simulink model "L_Trajectory_Tracking_and_Cartesian_Regulation"  (R2025b)
settings: Solver=FixedStepAuto  StartTime=0.0  StopTime=20.3895  FixedStep=Ts  RelTol=1e-3
values from neighbouring files (symbols this model uses):
  a = 50    [Lin_Traj_params.mat]    (also in automated_tuning_simulation.m = A_test(i); compare_methods.m = 15; simulation.m = 3; tuning_simulation.m = 15)
  Kv = 1    [Cartesian_gains.mat]    (also in simulation.m)
  Kw = 4    [Cartesian_gains.mat]    (also in simulation.m)
  shift_time = t(end)    [Plots.m]    (also in Plots_LvsNL.m; simulation.m; tuning_simulation.m)
  theta0 = -pi/2    (= -1.57079632679)    [automated_tuning_simulation.m]    (also in regulation_tuning_simulation.m = 0.785398163397; simulation.m = 0.785398163397; tuning_simulation.m = 0.785398163397)
  x0 = S.traj.xy(1,1)    [automated_tuning_simulation.m]    (also in regulation_tuning_simulation.m = -0.8; simulation.m; tuning_simulation.m)
  x_box = 850    [parking_box.mat]    (also in regulation_tuning_simulation.m = 0; replay_q_timeseries_on_maze_pacman.m; replay_q_timeseries_on_maze_pacman_real.m; simulation.m)
  xi = 0.7    [Lin_Traj_params.mat]    (also in NonLin_Traj_params.mat = 0.706; automated_tuning_simulation.m = XI_test(j); compare_methods.m = 0.706; simulation.m = 0.4)
  y0 = S.traj.xy(1,2)    [automated_tuning_simulation.m]    (also in regulation_tuning_simulation.m = 0.5; simulation.m; tuning_simulation.m)
  y_box = 880    [parking_box.mat]    (also in regulation_tuning_simulation.m = 0; replay_q_timeseries_on_maze_pacman.m; replay_q_timeseries_on_maze_pacman_real.m; simulation.m)
settings Model: Creator=emica  LastModifiedBy=emica
settings DataIOCC: ReturnWorkspaceOutputs=off

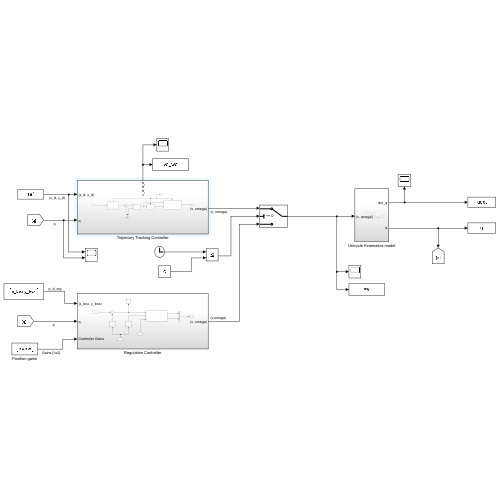
[thumbnail: Simulink's stored preview of the top-level diagram]
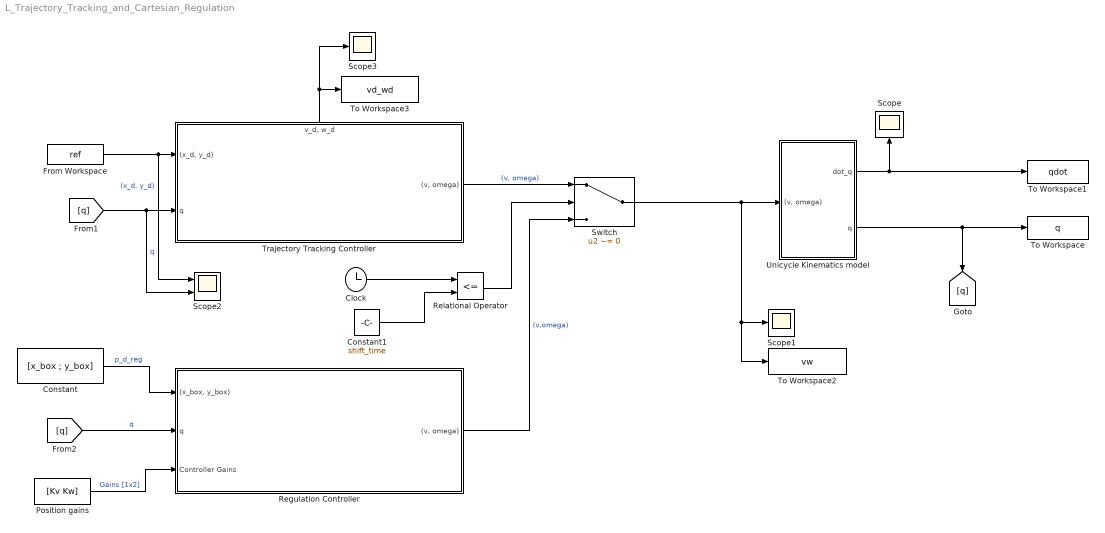
== system L_Trajectory_Tracking_and_Cartesian_Regulation ==
  Clock : Clock
  Constant : Constant  Value=[x_box ; y_box]
  Constant1 : Constant  Value=shift_time
  From Workspace : FromWorkspace  VariableName=ref  OutDataTypeStr=double  SampleTime=-1
  Position gains : Constant  Value=[Kv Kw]
  Regulation Controller : Subsystem
  Relational Operator : RelationalOperator  Operator=<=  OutDataTypeStr=boolean  RndMeth=Simplest  InputSameDT=off
  Scope : Scope
      settings: ActiveDisplayYMinimum=-404.1422156418318  ActiveDisplayYMaximum=218.29022715041242
  Scope1 : Scope
      settings: ActiveDisplayYMinimum=-533.5443121855302  ActiveDisplayYMaximum=284.37767608565741
  Scope2 : Scope  NumInputPorts=2
      settings: ActiveDisplayYMinimum=-357.06258853785005  ActiveDisplayYMaximum=1534.0761173534459  DataLoggingVariableName=ScopeData2
  Scope3 : Scope
      settings: ActiveDisplayYMinimum=-28.895296222010288  ActiveDisplayYMaximum=60.0576659980926  DataLoggingVariableName=ScopeData4
  Switch : Switch  Criteria=u2 ~= 0  Threshold=110  SaturateOnIntegerOverflow=off  InputSameDT=off
  To Workspace : ToWorkspace  VariableName=q  SaveFormat=Timeseries  SampleTime=-1
  To Workspace1 : ToWorkspace  VariableName=qdot  SaveFormat=Timeseries  SampleTime=-1
  To Workspace2 : ToWorkspace  VariableName=vw  SaveFormat=Timeseries  SampleTime=-1
  To Workspace3 : ToWorkspace  VariableName=vd_wd  SaveFormat=Timeseries  SampleTime=-1
  Trajectory Tracking Controller : Subsystem
      settings: PortSchema="{\"entries\":[{\"content\":{\"sides\":[{\"content\":{\"connectorIds\":[\"In1\",\"In2\"]},\"type\":\"ConnectorPlacement.EquallySpacedRectSide\",\"uuid\":\"cd877c46-8e15-457a-8f54-61807ea2ef45\"},{\"content\":{\"connectorIds\":[\"Out1\"],\"side\":\"RIGHT\"},\"type\":\"ConnectorPlacement.EquallySpacedRectSide\",\"uuid\":\"176f7bf5-d0a0-4212-99fa-33b58d1f7853\"},{\"content\":{\"connectorIds\":[\"Out2\"],\"side\":\"TOP\"},\"type\":\"ConnectorPlacement.EquallySpacedRectSide\",\"uuid\":\"ea12360e-3578-4fc6-8eb8-3473bdf68d44\"}]},\"type\":\"ConnectorPlacement.EquallySpacedConnector\",\"uuid\":\"d6941660-df06-4aa7-9a2d-244dac494f4a\"}],\"packageUris\":[\"http://schema.mathworks.com/mf0/Connector/R2020b\"],\"version\":\"1.0\"}"
  Unicycle Kinematics model : Subsystem
  wires:
  [q] -> Scope2/2, Trajectory Tracking Controller/2(q)  "q"
  Position gains/1 -> Regulation Controller/3(Controller Gains)  "Gains [1x2]"
  [q] -> Regulation Controller/2(q)  "q"
  Trajectory Tracking Controller/2("v_d, w_d") -> Scope3/1, To Workspace3/1
  Regulation Controller/1("(v, omega)") -> Switch/3  "(v,omega)"
  From Workspace/1 -> Scope2/1, Trajectory Tracking Controller/1("(x_d, y_d)")  "(x_d, y_d)"
  Constant1/1 -> Relational Operator/2
  Relational Operator/1 -> Switch/2
  Clock/1 -> Relational Operator/1
  Switch/1 -> To Workspace2/1, Scope1/1, Unicycle Kinematics model/1("(v, omega)")
  Trajectory Tracking Controller/1("(v, omega)") -> Switch/1  "(v, omega)"
  Unicycle Kinematics model/1(dot_q) -> To Workspace1/1, Scope/1
  Constant/1 -> Regulation Controller/1("(x_box, y_box)")  "p_d_reg"
  Unicycle Kinematics model/2(q) -> [q], To Workspace/1

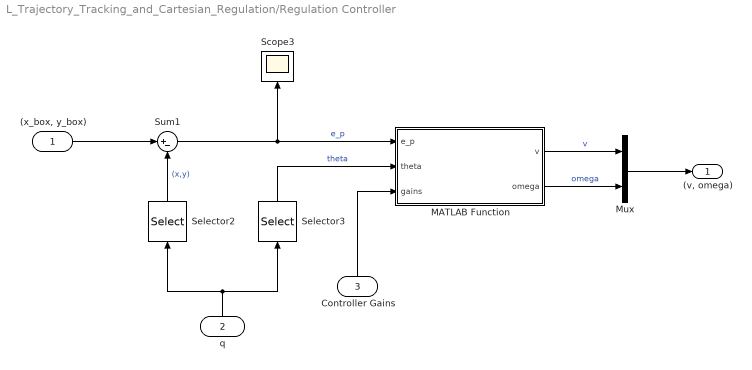
== system L_Trajectory_Tracking_and_Cartesian_Regulation/Regulation Controller ==
  "(x_box, y_box)" : Inport
  q : Inport  Port=2
  Controller Gains : Inport  Port=3
  MATLAB Function : MATLAB Function  TreatAsAtomicUnit=on
  Mux : Mux  Inputs=2
  Scope3 : Scope
      settings: ActiveDisplayYMinimum=-1.51842483246E+7  ActiveDisplayYMaximum=1.6973761395E+6  DataLoggingVariableName=ScopeData3
  Selector2 : Selector  InputPortWidth=3  IndexOptions=Index vector (dialog)  Indices=[1 2]  OutputSizes=1
  Selector3 : Selector  InputPortWidth=3  IndexOptions=Index vector (dialog)  Indices=[3]  OutputSizes=1
  Sum1 : Sum  Inputs=|+-
  "(v, omega)" : Outport
  wires:
  Selector2/1 -> Sum1/2  "(x,y)"
  Sum1/1 -> Scope3/1, MATLAB Function/1(e_p)  "e_p"
  Selector3/1 -> MATLAB Function/2(theta)  "theta"
  q/1 -> Selector3/1, Selector2/1
  Controller Gains/1 -> MATLAB Function/3(gains)
  "(x_box, y_box)"/1 -> Sum1/1
  MATLAB Function/1(v) -> Mux/1  "v"
  MATLAB Function/2(omega) -> Mux/2  "omega"
  Mux/1 -> "(v, omega)"/1

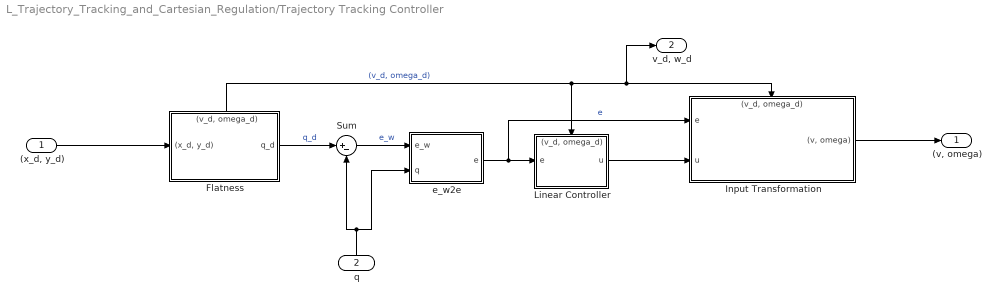
== system L_Trajectory_Tracking_and_Cartesian_Regulation/Trajectory Tracking Controller ==
  "(x_d, y_d)" : Inport
  q : Inport  Port=2
  Flatness : Subsystem
      settings: PortSchema="{\"entries\":[{\"content\":{\"sides\":[{\"content\":{\"connectorIds\":[\"In1\"]},\"type\":\"ConnectorPlacement.EquallySpacedRectSide\",\"uuid\":\"bc490c8e-5666-439b-9939-62bd84628b1f\"},{\"content\":{\"connectorIds\":[\"Out1\"],\"side\":\"RIGHT\"},\"type\":\"ConnectorPlacement.EquallySpacedRectSide\",\"uuid\":\"03a20fcc-2a82-4af2-a970-ff3426fda7d9\"},{\"content\":{\"connectorIds\":[\"Out2\"],\"side\":\"TOP\"},\"type\":\"ConnectorPlacement.EquallySpacedRectSide\",\"uuid\":\"09224fef-e39c-4959-bd2b-02867a510190\"}]},\"type\":\"ConnectorPlacement.EquallySpacedConnector\",\"uuid\":\"ad9510e9-14f7-413e-ab85-da35fb962608\"}],\"packageUris\":[\"http://schema.mathworks.com/mf0/Connector/R2020b\"],\"version\":\"1.0\"}"
  Input Transformation : Subsystem
      settings: PortSchema="{\"entries\":[{\"content\":{\"sides\":[{\"content\":{\"connectorIds\":[\"In1\",\"In2\"]},\"type\":\"ConnectorPlacement.EquallySpacedRectSide\",\"uuid\":\"4cbebdc1-8913-4bb0-9524-d854c819f784\"},{\"content\":{\"connectorIds\":[\"Out1\"],\"side\":\"RIGHT\"},\"type\":\"ConnectorPlacement.EquallySpacedRectSide\",\"uuid\":\"178a2b4a-0c33-47f3-8be3-bd76dfc47961\"},{\"content\":{\"connectorIds\":[\"In3\"],\"side\":\"TOP\"},\"type\":\"ConnectorPlacement.EquallySpacedRectSide\",\"uuid\":\"3e37ae07-0719-4d1d-ac53-f79374967c51\"}]},\"type\":\"ConnectorPlacement.EquallySpacedConnector\",\"uuid\":\"35111781-18f4-42cf-8750-882b65aa13c0\"}],\"packageUris\":[\"http://schema.mathworks.com/mf0/Connector/R2020b\"],\"version\":\"1.0\"}"
  Linear Controller : Subsystem
      settings: PortSchema="{\"entries\":[{\"content\":{\"sides\":[{\"content\":{\"connectorIds\":[\"In1\"]},\"type\":\"ConnectorPlacement.EquallySpacedRectSide\",\"uuid\":\"663a145a-b0a1-462d-957e-da25aa8d70ec\"},{\"content\":{\"connectorIds\":[\"Out1\"],\"side\":\"RIGHT\"},\"type\":\"ConnectorPlacement.EquallySpacedRectSide\",\"uuid\":\"3d00da72-66aa-4dae-9c0c-49820669bfbe\"},{\"content\":{\"connectorIds\":[\"In2\"],\"side\":\"TOP\"},\"type\":\"ConnectorPlacement.EquallySpacedRectSide\",\"uuid\":\"8e215669-d1a4-45b0-90e4-6e6fca69e90d\"}]},\"type\":\"ConnectorPlacement.EquallySpacedConnector\",\"uuid\":\"7b416759-2a96-476f-93d6-d6b19fa598e9\"}],\"packageUris\":[\"http://schema.mathworks.com/mf0/Connector/R2020b\"],\"version\":\"1.0\"}"
  Sum : Sum  Inputs=|+-
  e_w2e : MATLAB Function  TreatAsAtomicUnit=on
  "(v, omega)" : Outport
  "v_d, w_d" : Outport  Port=2
  wires:
  q/1 -> e_w2e/2(q), Sum/2
  Linear Controller/1(u) -> Input Transformation/2(u)
  e_w2e/1(e) -> Linear Controller/1(e), Input Transformation/1(e)  "e"
  Sum/1 -> e_w2e/1(e_w)  "e_w"
  Input Transformation/1("(v, omega)") -> "(v, omega)"/1
  Flatness/2("(v_d, omega_d)") -> Linear Controller/2("(v_d, omega_d)"), "v_d, w_d"/1, Input Transformation/3("(v_d, omega_d)")  "(v_d, omega_d)"
  Flatness/1(q_d) -> Sum/1  "q_d"
  "(x_d, y_d)"/1 -> Flatness/1("(x_d, y_d)")

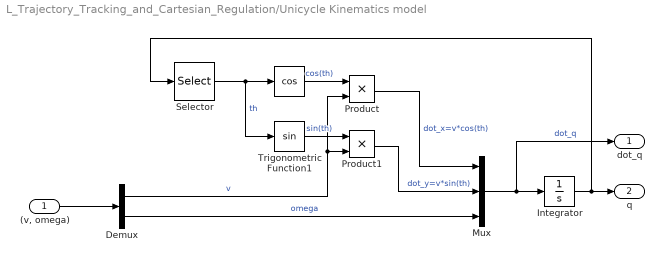
== system L_Trajectory_Tracking_and_Cartesian_Regulation/Unicycle Kinematics model ==
  "(v, omega)" : Inport
  " " : Trigonometry  Operator=cos
  Demux : Demux  Outputs=2
  Integrator : Integrator  InitialCondition=[x0; y0; theta0]
  Mux : Mux  Inputs=3
  Product : Product
  Product1 : Product
  Selector : Selector  InputPortWidth=3  IndexOptions=Index vector (dialog)  Indices=[3]  OutputSizes=1
  Trigonometric Function1 : Trigonometry
  dot_q : Outport
  q : Outport  Port=2
  wires:
  Integrator/1 -> Selector/1, q/1
  "(v, omega)"/1 -> Demux/1
  Mux/1 -> Integrator/1, dot_q/1  "dot_q"
  Demux/2 -> Mux/3  "omega"
  Selector/1 -> Trigonometric Function1/1, " "/1  "th"
  " "/1 -> Product/1  "cos(th)"
  Trigonometric Function1/1 -> Product1/1  "sin(th)"
  Demux/1 -> Product1/2, Product/2  "v"
  Product1/1 -> Mux/2  "dot_y=v*sin(th)"
  Product/1 -> Mux/1  "dot_x=v*cos(th)"

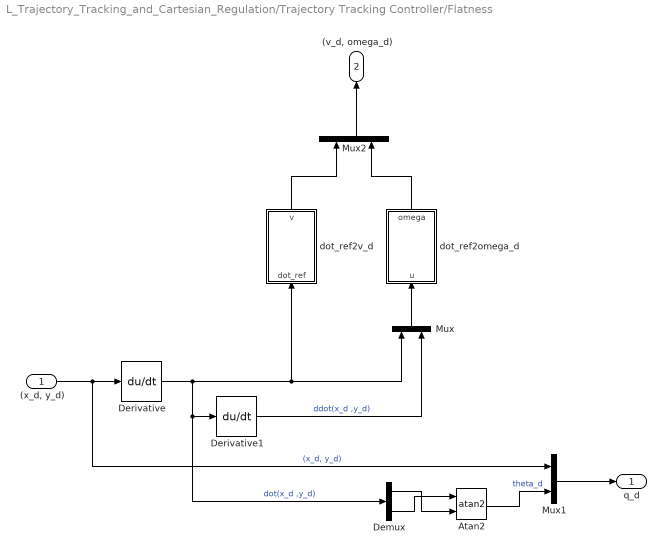
== system L_Trajectory_Tracking_and_Cartesian_Regulation/Trajectory Tracking Controller/Flatness ==
  "(x_d, y_d)" : Inport
  Atan2 : Trigonometry  Operator=atan2
  Demux : Demux  Outputs=2
  Derivative : Derivative
  Derivative1 : Derivative
  Mux : Mux  Inputs=2
  Mux1 : Mux  Inputs=2
  Mux2 : Mux  Inputs=2
  dot_ref2omega_d : MATLAB Function  TreatAsAtomicUnit=on
  dot_ref2v_d : MATLAB Function  TreatAsAtomicUnit=on
  q_d : Outport
  "(v_d, omega_d)" : Outport  Port=2
  wires:
  Atan2/1 -> Mux1/2  "theta_d"
  "(x_d, y_d)"/1 -> Mux1/1, Derivative/1  "(x_d, y_d)"
  Mux/1 -> dot_ref2omega_d/1(u)
  Derivative/1 -> Mux/1, dot_ref2v_d/1(dot_ref), Demux/1, Derivative1/1  "dot(x_d ,y_d)"
  Demux/1 -> Atan2/2
  Derivative1/1 -> Mux/2  "ddot(x_d ,y_d)"
  Demux/2 -> Atan2/1
  Mux1/1 -> q_d/1
  Mux2/1 -> "(v_d, omega_d)"/1
  dot_ref2omega_d/1(omega) -> Mux2/2
  dot_ref2v_d/1(v) -> Mux2/1

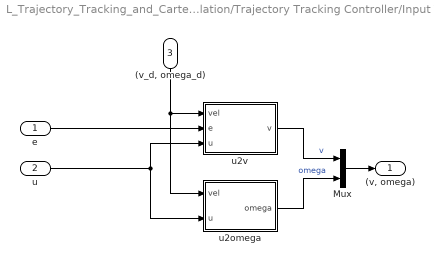
== system L_Trajectory_Tracking_and_Cartesian_Regulation/Trajectory Tracking Controller/Input Transformation ==
  e : Inport
  u : Inport  Port=2
  "(v_d, omega_d)" : Inport  Port=3
  Mux : Mux  Inputs=2
  u2omega : MATLAB Function  TreatAsAtomicUnit=on
  u2v : MATLAB Function  TreatAsAtomicUnit=on
  "(v, omega)" : Outport
  wires:
  e/1 -> u2v/2(e)
  Mux/1 -> "(v, omega)"/1
  u2omega/1(omega) -> Mux/2  "omega"
  u2v/1(v) -> Mux/1  "v"
  u/1 -> u2omega/2(u), u2v/3(u)
  "(v_d, omega_d)"/1 -> u2v/1(vel), u2omega/1(vel)

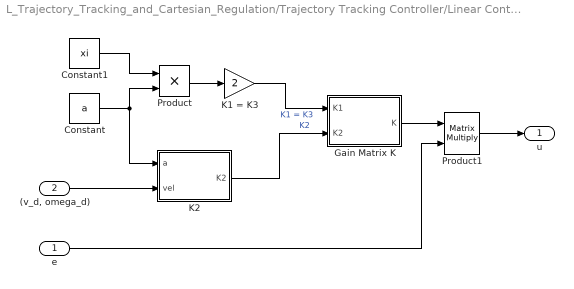
== system L_Trajectory_Tracking_and_Cartesian_Regulation/Trajectory Tracking Controller/Linear Controller ==
  e : Inport
  "(v_d, omega_d)" : Inport  Port=2
  Constant : Constant  Value=a
  Constant1 : Constant  Value=xi
  Gain Matrix K : MATLAB Function  TreatAsAtomicUnit=on
  K1 = K3 : Gain  Gain=2
  K2 : MATLAB Function  TreatAsAtomicUnit=on
  Product : Product
  Product1 : Product  Multiplication=Matrix(*)
  u : Outport
  wires:
  e/1 -> Product1/2
  Gain Matrix K/1(K) -> Product1/1
  Product1/1 -> u/1
  K2/1(K2) -> Gain Matrix K/2(K2)  "K2"
  K1 = K3/1 -> Gain Matrix K/1(K1)  "K1 = K3"
  Constant/1 -> K2/1(a), Product/2
  Constant1/1 -> Product/1
  "(v_d, omega_d)"/1 -> K2/2(vel)
  Product/1 -> K1 = K3/1

== matlab function L_Trajectory_Tracking_and_Cartesian_Regulation/Trajectory Tracking Controller/Flatness/dot_ref2omega_d ==
  data: u input; omega output
function omega = fcn(u)
    dot_x  = u(1);
    dot_y  = u(2);
    ddot_x = u(3);
    ddot_y = u(4);

    den = dot_x^2 + dot_y^2;

    % Guard against singularity / non-finite inputs
    eps_den = 1e-6;
    if ~isfinite(den) || den < eps_den
        omega = 0;             % safe default at standstill
        return;
    end

    num = dot_x*ddot_y - dot_y*ddot_x;

    if ~isfinite(num)
        omega = 0;
        return;
    end

    omega = num / den;

    % clamp extreme values
    omega_max = 20;            % rad/s
    if omega > omega_max
        omega = omega_max;
    elseif omega < -omega_max
        omega = -omega_max;
    end
end

== matlab function L_Trajectory_Tracking_and_Cartesian_Regulation/Trajectory Tracking Controller/Flatness/dot_ref2v_d ==
  data: dot_ref input; v output
function v = fcn(dot_ref)
    dot_x = dot_ref(1);
    dot_y = dot_ref(2);

    v = sqrt(dot_x^2 + dot_y^2);

    v_min = 1e-6;
    if ~isfinite(v) || v < v_min
        v = v_min;
    end
end

== matlab function L_Trajectory_Tracking_and_Cartesian_Regulation/Trajectory Tracking Controller/e_w2e ==
  data: e_w input; e output; q input
function e = fcn(e_w, q)
    theta = q(3);

    R = [cos(theta) sin(theta) 0; 
        -sin(theta) cos(theta) 0;
             0          0      1];

    e = R*e_w;

== matlab function L_Trajectory_Tracking_and_Cartesian_Regulation/Regulation Controller/MATLAB Function ==
  data: e_p input; v output; theta input; gains input; omega output
function [v, omega] = fcn(e_p, theta, gains)

Kv = gains(1);
Kw = gains(2);

v = Kv * ( e_p(1)*cos(theta) + e_p(2)*sin(theta) );

gamma = atan2(e_p(2), e_p(1)) + pi - theta;
gamma = atan2(sin(gamma), cos(gamma));  % to ensure that gamma in (-pi,pi)

omega = Kw * gamma;

== matlab function L_Trajectory_Tracking_and_Cartesian_Regulation/Trajectory Tracking Controller/Linear Controller/Gain Matrix K ==
  data: K1 input; K output; K2 input
function K = fcn(K1, K2)
K3 = K1;

K = [-K1  0   0;
      0  -K2 -K3];

== matlab function L_Trajectory_Tracking_and_Cartesian_Regulation/Trajectory Tracking Controller/Input Transformation/u2omega ==
  data: vel input; u input; omega output
function omega = fcn(vel,u)
    omega_d = vel(2);

    omega = omega_d-u(2);

== matlab function L_Trajectory_Tracking_and_Cartesian_Regulation/Trajectory Tracking Controller/Input Transformation/u2v ==
  data: vel input; e input; u input; v output
function v = fcn(vel, e, u)
 v_d = vel(1);

 v = v_d*cos(e(3))-u(1);

== matlab function L_Trajectory_Tracking_and_Cartesian_Regulation/Trajectory Tracking Controller/Linear Controller/K2 ==
  data: a input; vel input; K2 output
function K2 = fcn(a, vel)
v_d = vel(1);
omega_d = vel(2);

K2 = (a^2-omega_d^2)/(v_d);
